simulink model "VehicleModel_R2019a"  (R2019a)
settings: Solver=VariableStepAuto  StartTime=0.0  StopTime=10.0  RelTol=1e-3
libraries: simulink x2, vrlib x2
settings Model: Creator=yafta  LastModifiedBy=yafta

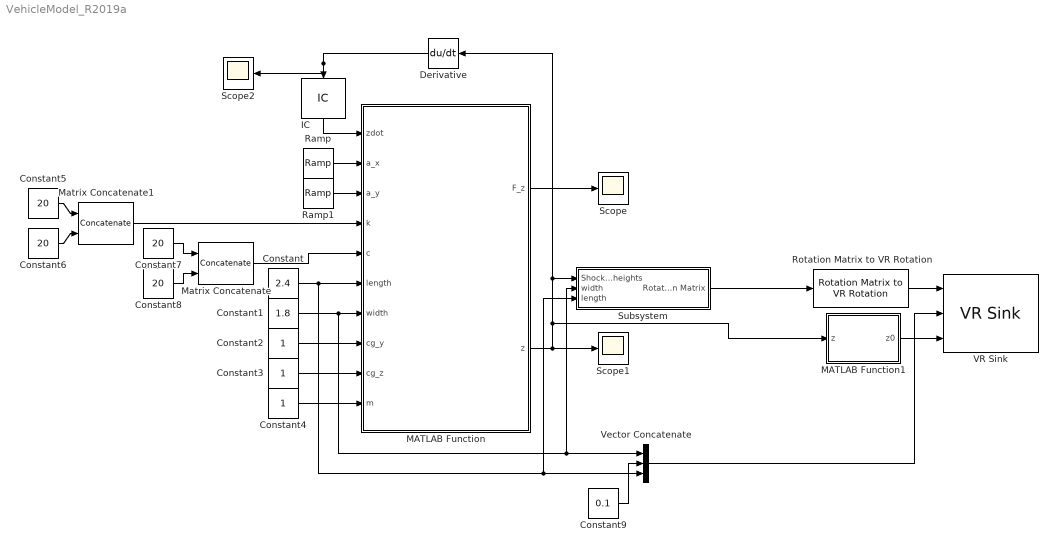
== system VehicleModel_R2019a ==
  Constant : Constant  Value=2.4
  Constant1 : Constant  Value=1.8
  Constant2 : Constant
  Constant3 : Constant
  Constant4 : Constant
  Constant{5..8} (4 alike) : Constant  Value=20
  Constant9 : Constant  Value=0.1
  Derivative : Derivative  CoefficientInTFapproximation=1
  IC : InitialCondition  Value=[1;1;1;1]
  MATLAB Function : MATLAB Function  TreatAsAtomicUnit=on
  MATLAB Function1 : MATLAB Function  TreatAsAtomicUnit=on
  Matrix Concatenate : Concatenate  Mode=Multidimensional array  ConcatenateDimension=2
  Matrix Concatenate1 : Concatenate  Mode=Multidimensional array  ConcatenateDimension=2
  Ramp : simulink/Sources/Ramp  slope=0.1  start=0  InitialOutput=0
  Ramp1 : simulink/Sources/Ramp  slope=0  start=0  InitialOutput=0
  Rotation Matrix to VR Rotation : vrlib/Utilities/Rotation Matrix to VR Rotation  maxzero=1e-12
      settings: SourceProductName=Simulink  SourceProductBaseCode=SL
  Scope : Scope
  Scope1 : Scope
  Scope2 : Scope
  Subsystem : Subsystem
  VR Sink : vrlib/VR Sink  InstantiateOnLoad=on  SampleTime=0.1  ViewEnable=on  RemoteChange=off  RemoteView=off  FieldsWritten=Box.rotation.4.1.1.double#Box.scale.3.1.1.double#Box.translation.3.1.1.double  WorldFileName=box.wrl  WorldDescription=Straight Road Strip - 2 Lanes  AutoView=off  VideoDimensions=[]  AllowVariableSize=off
      settings: SourceProductName=Simulink
  Vector Concatenate : Concatenate  NumInputs=3
  wires:
  MATLAB Function/2(z) -> MATLAB Function1/1(z), Derivative/1, Subsystem/1(Shock_heights), Scope1/1
  Derivative/1 -> Scope2/1, IC/1
  MATLAB Function/1(F_z) -> Scope/1
  Constant1/1 -> Subsystem/2(width), Vector Concatenate/1, MATLAB Function/7(width)
  Constant/1 -> Subsystem/3(length), Vector Concatenate/3, MATLAB Function/6(length)
  Constant2/1 -> MATLAB Function/8(cg_y)
  Constant3/1 -> MATLAB Function/9(cg_z)
  Constant4/1 -> MATLAB Function/10(m)
  Matrix Concatenate1/1 -> MATLAB Function/4(k)
  Matrix Concatenate/1 -> MATLAB Function/5(c)
  Constant5/1 -> Matrix Concatenate1/1
  Constant6/1 -> Matrix Concatenate1/2
  Constant7/1 -> Matrix Concatenate/1
  Constant8/1 -> Matrix Concatenate/2
  Ramp1/1 -> MATLAB Function/3(a_y)
  Ramp/1 -> MATLAB Function/2(a_x)
  IC/1 -> MATLAB Function/1(zdot)
  Constant9/1 -> Vector Concatenate/2
  Vector Concatenate/1 -> VR Sink/2
  Subsystem/1(Rotation Matrix) -> Rotation Matrix to VR Rotation/1
  MATLAB Function1/1(z0) -> VR Sink/3
  Rotation Matrix to VR Rotation/1 -> VR Sink/1

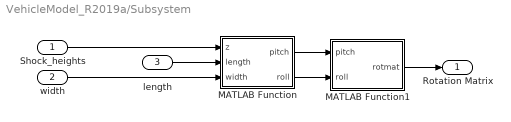
== system VehicleModel_R2019a/Subsystem ==
  Shock_heights : Inport
  width : Inport  Port=2
  length : Inport  Port=3
  MATLAB Function : MATLAB Function  TreatAsAtomicUnit=on
  MATLAB Function1 : MATLAB Function  TreatAsAtomicUnit=on
  Rotation Matrix : Outport
  wires:
  Shock_heights/1 -> MATLAB Function/1(z)
  MATLAB Function/1(pitch) -> MATLAB Function1/1(pitch)
  length/1 -> MATLAB Function/2(length)
  width/1 -> MATLAB Function/3(width)
  MATLAB Function1/1(rotmat) -> Rotation Matrix/1
  MATLAB Function/2(roll) -> MATLAB Function1/2(roll)

== matlab function VehicleModel_R2019a/Subsystem/MATLAB Function ==
  data: z input; pitch output; length input; width input; roll output
function [pitch, roll] = fcn(z, length, width)
avg_front = (z(1) + z(2))/2;
avg_rear = (z(3) + z(4))/2;
avg_left = (z(1) + z(3))/2;
avg_right = (z(2) + z(4))/2;
roll = atan((avg_right - avg_left)/width);
pitch = atan((avg_right - avg_rear)/length);

== matlab function VehicleModel_R2019a/MATLAB Function ==
  data: zdot input; F_z output; a_x input; a_y input; k input; c input; length input; width input; cg_y input; cg_z input; m input; z output
function [F_z,z] = verticalforces(zdot,a_x,a_y,k,c,length,width,cg_y,cg_z,m)
%     arguments
%         zdot (4,1) double   % Height rates of each wheel
%         a_x (1,1) double    % lateral (centripetal) acceleration
%         a_y (1,1) double    % longitudinal acceleration
%         k (2,1) double      % spring stiffnesses [front rear]
%         c (2,1) double      % damping coefficients [front rear]
%         length (1,1) double % distance from front to rear axle
%         width (1,1) double  % distance from left contact patch to right contact patch
%         cg_y (1,1) double   % forward distance from rear axle to CG
%         cg_z (1,1) double   % CG height from ground
%         m (1,1) double      % Vehicle mass
%     end
        % Calculate individual wheel vertical forces, heights and rates
A=[ 1,0,0,0,k(1),0,0,0;
    0,1,0,0,0,k(1),0,0;
    0,0,1,0,0,0,k(2),0;
    0,0,0,1,0,0,0,k(2);
    1,1,1,1,0,0,0,0;
    -cg_y,-cg_y,length-cg_y,length-cg_y,0,0,0,0;
    -width/2,width/2,-width/2,width/2,0,0,0,0;
    0,0,0,0,1,-1,-1,1];
b=[-zdot(1)*c(1);-zdot(2)*c(1);-zdot(3)*c(2);-zdot(4)*c(2);m*9.81;a_y*m*cg_z;a_x*m*cg_z;0];
x=A\b;
F_z=x(1:4);
z=x(5:8);
end

== matlab function VehicleModel_R2019a/MATLAB Function1 ==
  data: z input; z0 output
function z0 = translation(z)

z0=[0,-(z(1)+z(4))/2,0];

== matlab function VehicleModel_R2019a/Subsystem/MATLAB Function1 ==
  data: pitch input; rotmat output; roll input
function rotmat = fcn(pitch,roll)

rotmat = eul2rotm([0,pitch,roll]);
